simulink library "Lamp_Lib"  (R2022b)
settings: Solver=VariableStepAuto  StartTime=0.0  StopTime=10.0  RelTol=1e-3
undefined symbols (not defined in the file): APN_Param
libraries: spsThreePhaseSeriesRLCLoadLib x1, spsThreePhaseDynamicLoadLib x1
Description:
  | Copyright 2019-2022 The MathWorks, Inc.
settings Model: Creator=smiller  LastModifiedBy=smiller
settings SolverCC: AlgebraicLoopSolver=TrustRegion
settings DebuggingCC: UnconnectedInputMsg=warning  UnconnectedOutputMsg=warning  UnconnectedLineMsg=warning  SFMachineParentedDataDiag=warning
settings ModelReferenceCC: EnableRefExpFcnMdlSchedulingChecks=on
settings SFSimCC: CustomCodeUndefinedFunction=UseInterfaceOnly
settings RTWCC: DLArmComputeVersion=19.05

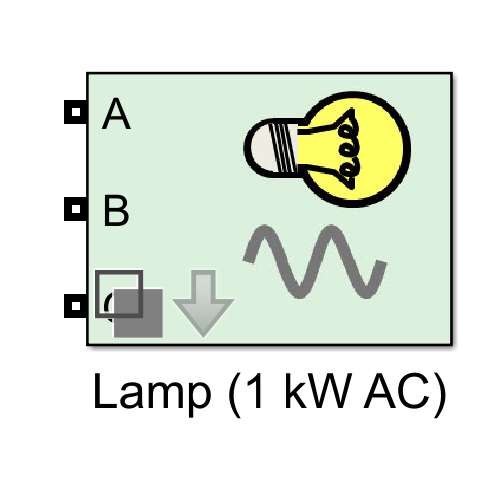
[thumbnail: Simulink's stored preview of the top-level diagram]
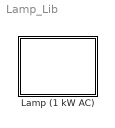
== system Lamp_Lib ==
  Lamp (1 kW AC) : Subsystem  RequirementInfo={} %GIDa_87e04d33_0159_4282_a5d2_2edb74190ab5  Variant=on  VariantControlMode=label  LabelModeActiveChoice=Detailed  mask{ModelType=Detailed, PQ_Model=Initial}
      mask prompts: ModelType "Model Type"; PQ_Model "PQ Model"
      mask init:
      | set_param(gcb,'LabelModeActiveChoice',get_param(gcb,'ModelType'));
      | set_param([gcb '/Phasor'],'PQ_Model',get_param(gcb,'PQ_Model'));
      settings: AttributesFormatString=%<BlockChoice>
      mask TypeOptions ModelType: Detailed | Phasor
      mask TypeOptions PQ_Model: Initial | Tuned
      mask Display:
      | blk = APN_activeVariantBlock(gcb);
      | eval(get_param(blk, 'MaskDisplay'));

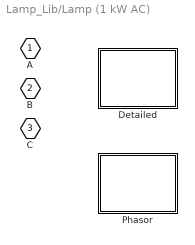
== system Lamp_Lib/Lamp (1 kW AC) ==
  Detailed : Subsystem  VariantControl=Detailed
      mask Display: image('LampAC_Detailed_IMAGE.jpg');
  Phasor : Subsystem  VariantControl=Phasor  mask{PQ_Model=Initial}
      mask prompts: PQ_Model "PQ Model"
      mask init:
      | set_param([gcb '/Calc PQ'],'PQ_Model',get_param(gcb,'PQ_Model'));
      mask TypeOptions PQ_Model: Initial | Tuned
      mask Display: image('LampAC_Phasor_IMAGE.jpg');
  A : PMIOPort  Side=Left
  B : PMIOPort  Port=2  Side=Left
  C : PMIOPort  Port=3  Side=Left

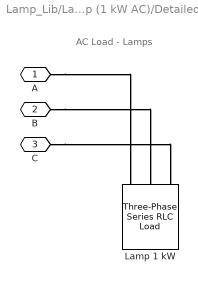
== system Lamp_Lib/Lamp (1 kW AC)/Detailed ==
  note: AC Load - Lamps
  Lamp 1 kW : spsThreePhaseSeriesRLCLoadLib/Three-Phase Series RLC Load  LConnTagsString=A|B|C  Configuration=Y (grounded)  NominalVoltage=200  Vabc=[1e3 1e3 1e3]  Vabcp=[1e3 1e3 1e3]  NominalFrequency=400  UnbalancedPower=off  ActivePower=1000  InductivePower=0  CapacitivePower=0  Pabc=[10e3 9e3 11e3]  QLabc=[100 90 110]  QCabc=[100 90 110]  Pabcp=[10e3 9e3 11e3]  QLabcp=[100 90 110]  QCabcp=[100 90 110]  Measurements=None  LoadType=constant Z
  A : PMIOPort  Side=Left
  B : PMIOPort  Port=2  Side=Left
  C : PMIOPort  Port=3  Side=Left
  connections:
  C/RConn1 -- Lamp 1 kW/LConn3
  B/RConn1 -- Lamp 1 kW/LConn2
  A/RConn1 -- Lamp 1 kW/LConn1

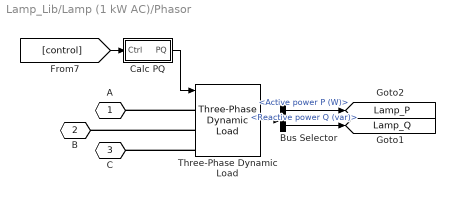
== system Lamp_Lib/Lamp (1 kW AC)/Phasor ==
  Bus Selector : BusSelector  OutputSignals=Active power P (W),Reactive power Q (var)
  Calc PQ : Subsystem  Variant=on  VariantControlMode=label  LabelModeActiveChoice=Initial  mask{PQ_Model=Initial}
      mask prompts: PQ_Model "PQ Model"
      mask init:
      | set_param(gcb,'LabelModeActiveChoice',get_param(gcb,'PQ_Model'));
      settings: AttributesFormatString=%<LabelModeActiveChoice>
      mask TypeOptions PQ_Model: Initial | Tuned
      mask Display: disp(' ')
  Three-Phase Dynamic Load : spsThreePhaseDynamicLoadLib/Three-Phase Dynamic Load  NominalVoltage=[ 200 400 ]  ActiveReactivePowers=[APN_Param.Lamp.P APN_Param.Lamp.Q]*0  PositiveSequence=[0.0004 0]  ExternalControl=on  NpNq=[1.3 2]  TimeConstants="[0  0  0  0]"  MinimumVoltage=0.7  Tfilter=1e-4  LoadFlowParameters=[4 0 0 0 0]
  A : PMIOPort  Side=Left
  B : PMIOPort  Port=2  Side=Left
  C : PMIOPort  Port=3  Side=Left
  tag scope: Lamp_P=global, Lamp_Q=global
  wires:
  Calc PQ/1(PQ) -> Three-Phase Dynamic Load/1
  [control] -> Calc PQ/1(Ctrl)
  Bus Selector/2 -> [Lamp_Q]  "<Reactive power Q (var)>"
  Three-Phase Dynamic Load/1 -> Bus Selector/1
  Bus Selector/1 -> [Lamp_P]  "<Active power P (W)>"
  connections:
  Three-Phase Dynamic Load/LConn1 -- A/RConn1
  Three-Phase Dynamic Load/LConn2 -- B/RConn1
  Three-Phase Dynamic Load/LConn3 -- C/RConn1

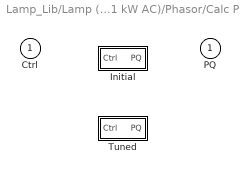
== system Lamp_Lib/Lamp (1 kW AC)/Phasor/Calc PQ ==
  Ctrl : Inport
  Initial : Subsystem  VariantControl=Initial
  Tuned : Subsystem  VariantControl=Tuned
  PQ : Outport  VectorParamsAs1DForOutWhenUnconnected=off

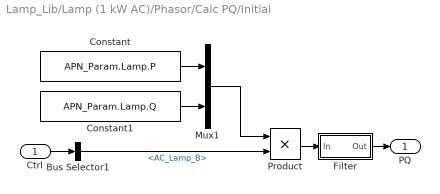
== system Lamp_Lib/Lamp (1 kW AC)/Phasor/Calc PQ/Initial ==
  Ctrl : Inport
  Bus Selector1 : BusSelector  OutputSignals=AC_Lamp_B
  Constant : Constant  Value=APN_Param.Lamp.P
  Constant1 : Constant  Value=APN_Param.Lamp.Q
  Filter : Subsystem  mask(First-order lag supporting vector signals){b=1e-2, x_initial=[APN_Param.Lamp.P APN_Param.Lamp.Q]*0}
      mask prompts: b "Filter time constant"; x_initial "Initial output"
      mask help: Models a lag of the form 1/(b*s+1) where s is the Laplace operator.
  Mux1 : Mux  Inputs=2
  Product : Product
  PQ : Outport  VectorParamsAs1DForOutWhenUnconnected=off
  wires:
  Product/1 -> Filter/1(In)
  Constant1/1 -> Mux1/2
  Constant/1 -> Mux1/1
  Mux1/1 -> Product/1
  Filter/1(Out) -> PQ/1
  Bus Selector1/1 -> Product/2  "<AC_Lamp_B>"
  Ctrl/1 -> Bus Selector1/1

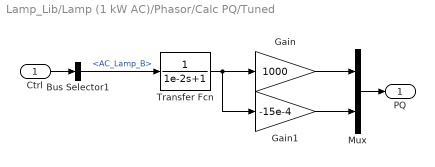
== system Lamp_Lib/Lamp (1 kW AC)/Phasor/Calc PQ/Tuned ==
  Ctrl : Inport
  Bus Selector1 : BusSelector  OutputSignals=AC_Lamp_B
  Gain : Gain  Gain=1000
  Gain1 : Gain  Gain=-15e-4
  Mux : Mux  Inputs=2
  Transfer Fcn : TransferFcn  Denominator=[1e-2 1]
  PQ : Outport  VectorParamsAs1DForOutWhenUnconnected=off
  wires:
  Ctrl/1 -> Bus Selector1/1
  Bus Selector1/1 -> Transfer Fcn/1  "<AC_Lamp_B>"
  Gain1/1 -> Mux/2
  Gain/1 -> Mux/1
  Transfer Fcn/1 -> Gain/1, Gain1/1
  Mux/1 -> PQ/1

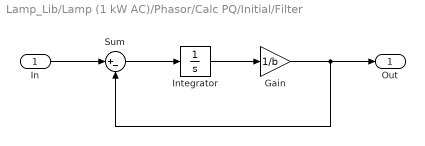
== system Lamp_Lib/Lamp (1 kW AC)/Phasor/Calc PQ/Initial/Filter ==
  In : Inport
  Gain : Gain  Gain=1/b
  Integrator : Integrator  InitialCondition=x_initial
  Sum : Sum  Inputs=|+-  InputSameDT=on  SaturateOnIntegerOverflow=on  OutDataTypeStr=Inherit: Same as first input
  Out : Outport  VectorParamsAs1DForOutWhenUnconnected=off
  wires:
  Sum/1 -> Integrator/1
  In/1 -> Sum/1
  Integrator/1 -> Gain/1
  Gain/1 -> Sum/2, Out/1
